simulink model "TRN_V3_CodeGen"  (R2022a)
settings: Solver=FixedStepAuto  StartTime=0.0  StopTime=300  FixedStep=0.04  RelTol=1e-3
PreLoadFcn:
  | % Add DataBus Path
  | addpath(',/TRN');
  | addpath('./MAP/');
  | addpath('./MAP/MAP_DB');
  | addpath('./MAP/DVOF');
  | addpath(genpath(cd));
  | load('BusStructureTRN.mat');
InitFcn:
  | % Add DataBus Path
  | addpath(',/TRN');
  | addpath('./MAP/');
  | addpath('./MAP/MAP_DB');
  | addpath('./MAP/DVOF');
  | addpath(genpath(cd));
  | load('BusStructureTRN.mat');
undefined symbols (not defined in the file or in its folder): Altitude_INS, INSDataNotValid, Latitude_INS, Longitude_INS, RALTValid, TRN, TRNlib
libraries: simulink_extras x33, aerolibconvert2 x6, dspstat3 x3, sharedtransform x2
(part 3 of 3)

== matlab function TRN_V3_CodeGen/TRN/INS//GPSFilter/MesurementUpdate Function ==
  data: Lat_GPS input; Hmatrix output; Lon_GPS input; z output; alt_GPS input; velN_GPS input; velE_GPS input; velD_GPS input; Lat_INS input; Lon_INS input; alt_INS input; velN_INS input; velE_INS input; velD_INS input; M input; N input; psi input
function [Hmatrix, z] = MeasurementUpdate(Lat_GPS, Lon_GPS, alt_GPS, velN_GPS, velE_GPS, velD_GPS, ...
                                          Lat_INS, Lon_INS, alt_INS, velN_INS, velE_INS, velD_INS, ...
                                          M, N, psi)

alt = alt_INS;

Z   = zeros(3);
I   = eye(3);
H   = [(M+alt)        0             0;
         0     (N+alt)*cos(psi)     0;
         0            0             1;];

% H matrix
Hmatrix = [ H Z Z
            Z I Z]; 

z = [(M+alt)*(Lat_INS-Lat_GPS); 
    (N+alt)*cos(psi)*(Lon_INS-Lon_GPS);
     alt_INS - alt_GPS;
    velN_INS - velN_GPS;
    velE_INS - velE_GPS;
    velD_INS - velD_GPS;];


end

== matlab function TRN_V3_CodeGen/TRN/INS//GPSFilter/MesurementUpdate Function1 ==
  data: M output; N output; psi output; in_psi input
function [M, N, psi] = Earth_radius(in_psi)

    a   = 6378137;          % Earth's equatorial radius
    b   = 6356752.314245;   % Earth's polar radius
    psi = in_psi;           % psi(latitude_GPS)
    M   = ((a*b)^2) / ( ( (a*cos(psi))^2 + (b*sin(psi))^2 )^(3/2) );    % radius  of  curvature  in  meridian
    N   = (a^2) / ( ( (a*cos(psi))^2 + (b*sin(psi))^2 )^(1/2) );        % radius  of  curvature  in  prime  vertical

end

== matlab function TRN_V3_CodeGen/TRN/INS//GPSFilter/MesurementUpdate Function2 ==
  data: Lat_LCI output; Lat_INS input; Lon_INS input; alt_INS input; Lon_LCI output; alt_LCI output; Lat_LCI input; Lon_LCI input; alt_LCI input
function [Lat_LCI, Lon_LCI, alt_LCI] = MeasurementUpdate(Lat_INS, Lon_INS, alt_INS, ...
                                                                      Lat_LCI, Lon_LCI, alt_LCI)
    Lat_LCI = Lat_INS  - Lat_LCI;
    Lon_LCI = Lon_INS  - Lon_LCI;
    alt_LCI = alt_INS  - alt_LCI;

end

== matlab function TRN_V3_CodeGen/TRN/INS//GPSFilter/Rupdate Function ==
  data: Lat_GPS input; Rmatrix output; Lon_GPS input; alt_GPS input; velN_GPS input; velE_GPS input; velD_GPS input
% ---------------------------------------------------------------------- %
%                   R matrix update function
% ---------------------------------------------------------------------- %
function Rmatrix = Rupdate(Lat_GPS, Lon_GPS, alt_GPS, velN_GPS, velE_GPS, velD_GPS)

%     Rmatrix = diag([ std(Lat_GPS)^2 std(Lon_GPS)^2 std(alt_GPS)^2 std(velN_GPS)^2 std(velE_GPS)^2 std(velD_GPS)^2 ]);
%     Rmatrix = diag([ (6.6/sqrt(25))^2 (6.6/sqrt(25))^2 (6.6/sqrt(25))^2 (6.6/sqrt(25))^2 (6.6/sqrt(25))^2 (6.6/sqrt(25))^2 ]);
    Rmatrix = diag([ (6.6/sqrt(25))^2 (6.6/sqrt(25))^2 (1/sqrt(25))^2 (0.5/sqrt(25))^2 (0.5/sqrt(25))^2 (0.5/sqrt(25))^2 ]);
%     Rmatrix = diag([ (6.6/sqrt(25))^2 (6.6/sqrt(25))^2 (6.6/sqrt(25))^2 (0.0)^2 (0.0)^2 (0.0)^2 ]);

end

== matlab function TRN_V3_CodeGen/TRN/TRNSchedulerDTNS1/TrackingCSU/TrackingCSU1/EKFupdate/EKFUpdate Function ==
  data: z input; xu output; xp output; P output; F input; H input; G input; P input; Q input; R input; dt input; residual output; latINSErrTRN output; lonINSErrTRN output; altINSErrTRN output; hUncertainty output; vUncertainty output; xu_prev input; TimeTag input
function [xu, xp, P, residual, latINSErrTRN, lonINSErrTRN, altINSErrTRN, ...
          hUncertainty, vUncertainty] = EKFUpdate(z, F, H, G, P, Q, R, dt, xu_prev, TimeTag)

x = zeros(15,1);
I = eye(max(size(F)));

A = I + (F*dt);
Q = (A*G * Q * G'*A') .* dt;

%-------------------------------------%
% Predicts states & covariance matrix
%-------------------------------------%
xp = A * x;
Pp = (A * P * A') + Q;

%---------------------%
% Updates Kalman gain
%---------------------%
K = (Pp * H')/(R + H * Pp * H');

%----------------%
% Updates states
%----------------%
xu = xp + K * (z - H*xp);
% residual = z - H*xp;
residual = z;

%---------------------------%
% Updates covariance matrix
%---------------------------%
P = (I - K*H) * Pp * (I - K*H)' + K*R*K';


latINSErrTRN = xu(7);
lonINSErrTRN = xu(8);
altINSErrTRN = xu(9);
hUncertainty = sqrt(abs(P(7,7) + P(8,8)));
vUncertainty = sqrt(abs(P(9,9)));
AGLErrTRN    = uint16(vUncertainty+ sqrt(R)*randn(1));

if TimeTag(6) == 1
    xu = xu_prev;
    latINSErrTRN = xu(7);
    lonINSErrTRN = xu(8);
    altINSErrTRN = xu(9);
end

end

== matlab function TRN_V3_CodeGen/TRN/TRNSchedulerDTNS1/TrackingCSU/TrackingCSU1/Measurement/Fupdate Function ==
  data: velN input; Fmatrix output; velE input; velD input; lat input; alt input; accN input; accE input; accD input; OM input; R0 input; DCMbn input; M input; N input
% ---------------------------------------------------------------------- %
%                   F matrix update function
%
%   INPUT:
%       velN: North Velocity                                [m/s]
%       velE: East Velocity                                 [m/s]
%       velD: Down Velocity                                 [m/s]
%       lat: Latitude                                       [rad]
%       alt: Altitude                                       [m]
%       accN: North acceleration                            [m/ss]
%       accE: East acceleration                             [m/ss]
%       accD: Down acceleration                             [m/ss]
%       OM: Magnitude of the rotation rate of the Earth     [rad/s]
%       R0: Radius of Earth                                 [m]
%       DCMbn: Rotational matrix(body frame to navigation frame)
%
%   OUTPUT:
%       Fmatrix: System matrix of Kalman Filter
%
% ---------------------------------------------------------------------- %
function Fmatrix = Fupdate(velN, velE, velD, lat, alt, accN, accE, accD, OM, R0, DCMbn, M, N)
    
        Z  = zeros(3);
    
        e11 = 0;
        e12 = -((OM * sin(lat)) + (velE/(N+alt) * tan(lat)));
        e13 = velN/(M+alt);
        e21 = ((OM * sin(lat)) + (velE/(N+alt) * tan(lat)));
        e22 = 0;
        e23 = ((OM * cos(lat)) + (velE/(N+alt)));
        e31 = -velN/(M+alt);
        e32 = -(OM * cos(lat)) - (velE/(N+alt));
        e33 = 0;
        Fee = [e11 e12 e13; e21 e22 e23; e31 e32 e33;];
    
        e11 = 0;
        e12 = 1/((N+alt));
        e13 = 0;
        e21 = -1/((M+alt));
        e22 = 0 ;
        e23 = 0 ;
        e31 = 0 ;
        e32 = -tan(lat)/(N+alt) ;
        e33 = 0 ;
        Fev = [e11 e12 e13; e21 e22 e23; e31 e32 e33;];
    
        e11 = -OM * sin(lat);
        e12 = 0;
        e13 = -velE/(((N+alt))^2);
        e21 = 0 ;
        e22 = 0 ;
        e23 = velN/(((M+alt))^2);
        e31 =  -(OM*cos(lat)) - (velE/(((N+alt))*(cos(lat))^2));
        e32 = 0 ;
        e33 = (velE * tan(lat)) / ((N+alt)^2) ;
        Fep = [e11 e12 e13; e21 e22 e23; e31 e32 e33;];
    
        e11 = 0 ;
        e12 = -accD ;
        e13 = accE ;
        e21 = accD ;
        e22 = 0 ;
        e23 = -accN ;
        e31 = -accE ;
        e32 = accN ;
        e33 = 0 ;
        Fve = [e11 e12 e13; e21 e22 e23; e31 e32 e33;];
    
        e11 = velD/((M+alt));
        e12 = -2*((OM * sin(lat)) + ((velE/((N+alt))) * tan (lat))) ;
        e13 = velN/(M+alt) ;
        e21 = (2*OM * sin(lat)) + ( (velE/((N+alt))) * tan(lat) );
        e22 = (1/((N+alt))) * ((velN * tan(lat)) + velD) ;
        e23 = 2*OM * cos(lat) + (velE/((N+alt)));
        e31 = (-2*velN)/((M+alt));
        e32 = -2*(OM * cos(lat) +  (velE/((N+alt)))) ;
        e33 = 0;
        Fvv = [e11 e12 e13; e21 e22 e23; e31 e32 e33;];
    
        e11 = -velE*( (2*OM * cos(lat)) + (velE/(((N+alt))*(cos(lat))^2)));
        e12 = 0 ;
        e13 = (((velE^2)*tan(lat))/((N+alt)^2)) - ((velN*velD)/((M+alt)^2)) ;
        e21 = 2*OM *((velN*cos(lat)) - (velD*sin(lat))) + ((velN*velE) / (((N+alt))*(cos(lat))^2)) ;
        e22 = 0 ;
        e23 = ((-velE*velD)/((N+alt)^2))-((velN*velE*tan(lat))/((N+alt)^2));
        e31 = 2 * OM * velE * sin(lat);
        e32 = 0;
        e33 =  (((velE^2)/((N+alt)^2)) + ((velN^2)/((M+alt)^2)));
        Fvp = [e11 e12 e13; e21 e22 e23; e31 e32 e33;];
    
        Fpe = zeros(3);
    
        e11 = 1/((M+alt));
        e12 = 0;
        e13 = 0;
        e21 = 0;
        e22 = 1/(((N+alt))*cos(lat));
        e23 = 0;
        e31 = 0;
        e32 = 0;
        e33 = -1;
        Fpv = [e11 e12 e13; e21 e22 e23; e31 e32 e33;];
    
        e11 = 0;
        e12 = 0;
        e13 = -velN/(((M+alt))^2);
        e21 = (velE*tan(lat))/(((N+alt))*cos(lat));
        e22 = 0;
        e23 = -velE/((((N+alt))^2)*cos(lat));
        e31 = 0;
        e32 = 0;
        e33 = 0;
        Fpp = [e11 e12 e13; e21 e22 e23; e31 e32 e33;];
    
    
        %     Fvv = zeros(3);
        %     Fvp = zeros(3);
        %     Fpp = zeros(3);
    
        Fmatrix =  [Fee    Fev    Fep      DCMbn          Z      ;
                    Fve    Fvv    Fvp        Z           DCMbn   ;
                    Fpe    Fpv    Fpp        Z            Z      ;
                    Z      Z      Z          Z            Z      ;
                    Z      Z      Z          Z            Z      ;];


end

== matlab function TRN_V3_CodeGen/TRN/TRNSchedulerDTNS1/TrackingCSU/TrackingCSU1/Measurement/Gupdate Function ==
  data: DCMbn input; Gmatrix output
% ---------------------------------------------------------------------- %
%                   G matrix update function
%
%   INPUT:
%       DCMbn: Rotational matrix(body frame to navigation frame)
%
%   OUTPUT:
%       Gmatrix: Input matrix of Kalman Filter
%
% ---------------------------------------------------------------------- %
function Gmatrix = Gupdate(DCMbn)

Z  = zeros(3);
I  = eye(3);

Gmatrix =  [ -DCMbn     Z;
                Z      DCMbn;
                Z       Z;
                Z       Z;
                Z       Z;];      

end

== matlab function TRN_V3_CodeGen/TRN/TRNSchedulerDTNS1/TrackingCSU/TrackingCSU1/Measurement/MATLAB Function1 ==
  data: RALTValid input; roll input; pitch input; z_out output; z_in input
function z_out = fcn(RALTValid, roll, pitch, z_in)

z_out = 0;

if RALTValid == true && abs(roll) < deg2rad(15) && abs(pitch) < deg2rad(15)
    z_out = z_in;

else
    z_out = 0;
end

== matlab function TRN_V3_CodeGen/TRN/TRNSchedulerDTNS1/TrackingCSU/TrackingCSU1/Measurement/MesurementUpdate Function ==
  data: Hmatrix output; lat input; lon input; alt input; RALT input; z output
% function [Hmatrix, z, hDEM] = MeasurementUpdate(resolution, lat, lon, alt, RALT)
function [Hmatrix, z] = MeasurementUpdate(lat, lon, alt, RALT)

%% DTRAN
%     P11 = 0;
%     P12 = 0;    
%     P21 = 0;    
%     P22 = 0;
%     
%     x = mod( (lon - leftLon)/resolution, 1 )*resolution;  y = mod( (lat - bottomLat)/resolution, 1)*resolution;
%     
%     leftLonIndex   =   floor( (lon - leftLon)/resolution );
%     lowerLatIndex  =   floor( (lat - bottomLat)/resolution );
%     
%     P11 = coder.ceval('GetElevationFromIndex', lowerLatIndex, leftLonIndex);
%     P12 = coder.ceval('GetElevationFromIndex', lowerLatIndex, leftLonIndex+1);
%     P21 = coder.ceval('GetElevationFromIndex', lowerLatIndex+1, leftLonIndex);
%     P22 = coder.ceval('GetElevationFromIndex', lowerLatIndex+1, leftLonIndex+1);
%     
%     if P11 < -12000 || P11 > 9000
%         P11 = 0;
%     end
%     if P12 < -12000 || P12 > 9000
%         P12 = 0;
%     end
%     if P21 < -12000 || P21 > 9000
%         P21 = 0;
%     end
%     if P22 < -12000 || P22 > 9000
%         P22 = 0;
%     end
%     
%     P_low    =   (resolution-x)/resolution * P11    +   (x/resolution) * P12;
%     P_high   =   (resolution-x)/resolution * P21    +   (x/resolution) * P22;
%     P_left   =   (resolution-y)/resolution * P11    +   (y/resolution) * P21;
%     P_right  =   (resolution-y)/resolution * P12    +   (y/resolution) * P22;
%     
%     hdot_lat    =   (P_high - P_low) / resolution;
%     hdot_lon    =   (P_right - P_left) / resolution;
%     
%     % H matrix
%     Hmatrix     =  [ zeros(1,6) -hdot_lat   -hdot_lon    1  zeros(1,6) ]; 
%     
%     hDEM = (resolution-y)/resolution * P_low  +   (y/resolution) * P_high;
%     
%     z = (alt - hDEM) - RALT;

%% DTNS
    P_low = 0.0;
    P_high = 0.0;    
    P_left = 0.0;    
    P_right = 0.0;
    hDEM = double(0.0);         
    resultDTED = uint32(1);
    resultDVOF = int32(1);

    resolution = 3 * 0.000277777777777777;

    lat = rad2deg(lat);
    lon = rad2deg(lon);
    
    resultDVOF = coder.ceval('UpdateObstList', lat, lon);
    resultDTED = coder.ceval('UpdateMapCache', lat, lon);
    
    P_low    =   coder.ceval('GetElevation', lat - resolution, lon);
    P_high   =   coder.ceval('GetElevation', lat + resolution, lon);
    P_left   =   coder.ceval('GetElevation', lat, lon - resolution);
    P_right  =   coder.ceval('GetElevation', lat, lon + resolution);
    
    hdot_lat    =   (P_high - P_low) / resolution;
    hdot_lon    =   (P_right - P_left) / resolution;
    
    % H matrix
    Hmatrix     =  [ zeros(1,6) -hdot_lat   -hdot_lon    1  zeros(1,6) ]; 
    
    hDEM = coder.ceval('GetElevation', lat, lon);
    
    z = (alt - hDEM) - RALT;

end

== matlab function TRN_V3_CodeGen/TRN/INS//GPSFilter/MATLAB Function1 ==
  data: GPSValid input; z_out output; z_in input; Lat_GPS input; Lat_GPS_temp input; Lon_GPS input; Lon_GPS_temp input
function z_out = fcn(GPSValid, z_in, Lat_GPS, Lat_GPS_temp, Lon_GPS, Lon_GPS_temp)

z_out = zeros(6,1);

if GPSValid == 0    % GPS valid
    if (abs(rad2deg(Lat_GPS - Lat_GPS_temp)) < 0.000000001) || (abs(rad2deg(Lon_GPS - Lon_GPS_temp)) < 0.000000001)    % Propagation  
        z_out = zeros(6,1);
    else                % Update
        z_out = z_in;
    end   
    
else
    z_out = zeros(6,1);
end

== matlab function TRN_V3_CodeGen/TRN/INS//GPSFilter/ConvertINSInput/MATLAB Function2 ==
  data: TimeTag_Prev input; TimeTag_Prev output; GPSTimeTag input; INSTimeTag input; RALTTimeTag input
function TimeTag_Prev   = fcn(TimeTag_Prev,GPSTimeTag,INSTimeTag,RALTTimeTag)


TimeTag_Prev(4) = 0;
TimeTag_Prev(5) = 0;
TimeTag_Prev(6) = 0;

if TimeTag_Prev(1) == GPSTimeTag
    TimeTag_Prev(4) = 1;
end

if TimeTag_Prev(2) == INSTimeTag
    TimeTag_Prev(5) = 1;
end

if TimeTag_Prev(3) == RALTTimeTag
    TimeTag_Prev(6) = 1;
end

TimeTag_Prev(1) = GPSTimeTag;
TimeTag_Prev(2) = INSTimeTag;
TimeTag_Prev(3) = RALTTimeTag;

== matlab function TRN_V3_CodeGen/TRN/TRNSchedulerDTNS1/TrackingCSU/TrackingCSU1/EKFupdate/MATLAB Function1 ==
  data: u input; y1 output; y2 output; y3 output
function [y1,y2,y3] = fcn(u)
    y = (u);
    yy = [y(7), y(8), y(9)];
    utm_lat2m_deg = 110961.7060516;   
    utm_lon2m_deg = 89476.51124;

    y1 = rad2deg(yy(1))*utm_lat2m_deg;
    y2 = rad2deg(yy(2))*utm_lon2m_deg;
    y3 = yy(3);

end
